simulink library "Surface_Profile_Axle2_zx_LR"  (R2025a)
settings: Solver=VariableStepAuto  StartTime=0.0  StopTime=10.0  RelTol=1e-3
Description:
  | Simscape Vehicle Templates Library
  | 
  | Copyright 2018-2025 The MathWorks, Inc.
settings Model: Creator=smiller  LastModifiedBy=smiller
settings ModelReferenceCC: EnableRefExpFcnMdlSchedulingChecks=on
settings RTWCC: GPUComputeCapability=3.5

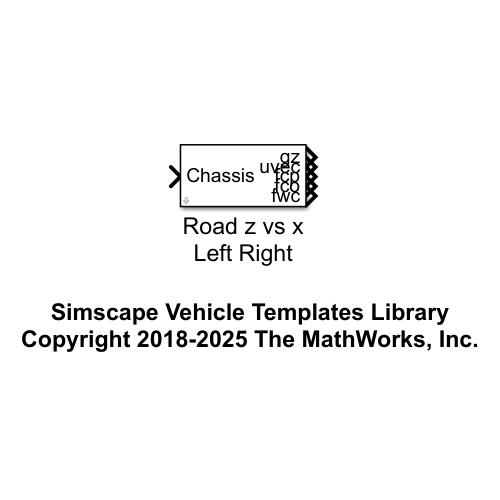
[thumbnail: Simulink's stored preview of the top-level diagram]
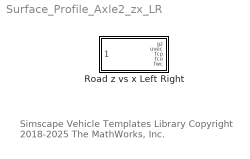
== system Surface_Profile_Axle2_zx_LR ==
  note: Simscape Vehicle Templates Library
      | Copyright 2018-2025 The MathWorks, Inc.
  Road z vs x Left Right : Subsystem  VariantControl=Rough_Road  mask{dist_x_l=flipud(Scene.RDF_Rough_Road.Road.extr_data_L(1330:end,1)), height_z_l=flipud(Scene.RDF_Rough_Road.Road.extr_data_L(1330:end,2)), dist_x_r=flipud(Scene.RDF_Rough_Road.Road.extr_data_R(1330:end,1)), height_z_r=flipud(Scene.RDF_Rough_Road.Road.extr_data_R(1330:end,2))}
      mask prompts: dist_x_l "Distance Vector Left [x] (m)"; height_z_l "Height Vector Left [z] (m)"; dist_x_r "Distance Vector Right [x] (m)"; height_z_r "Height Vector Right [z] (m)"
      mask init:
      | pitch_l = atan2(circshift(height_z_l,-2)-circshift(height_z_l,2),circshift(dist_x_l,-2)-circshift(dist_x_l,2));
      | pitch_l(1:2) = pitch_l(3);
      | pitch_l(end-1:end) = pitch_l(end-2);
      | 
      | pitch_r = atan2(circshift(height_z_r,-2)-circshift(height_z_r,2),circshift(dist_x_r,-2)-circshift(dist_x_r,2));
      | pitch_r(1:2) = pitch_r(3);
      | pitch_r(end-1:end) = pitch_r(end-2);

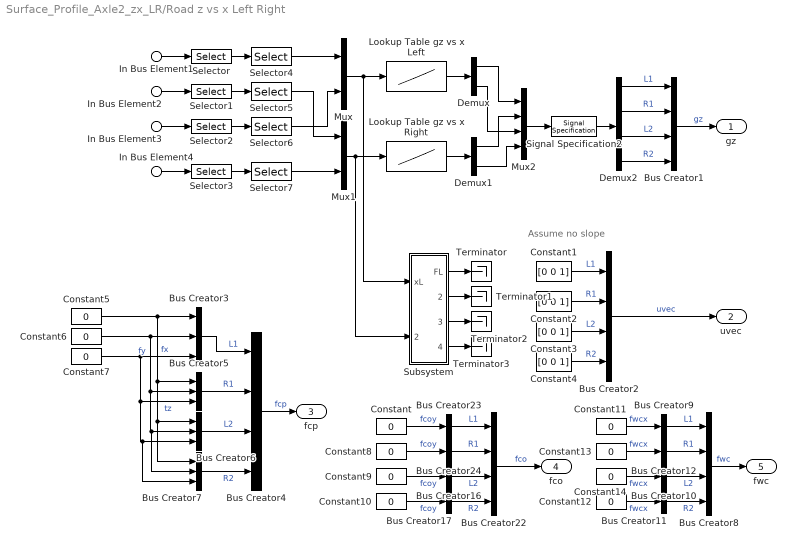
== system Surface_Profile_Axle2_zx_LR/Road z vs x Left Right ==
  note: Assume no slope
  In Bus Element1 : Inport  PortName=Chassis  Element=WhlL1.xyz
  In Bus Element2 : Inport  PortName=Chassis  Element=WhlR1.xyz
  In Bus Element3 : Inport  PortName=Chassis  Element=WhlL2.xyz
  In Bus Element4 : Inport  PortName=Chassis  Element=WhlR2.xyz
  Bus Creator{1..2,4,8,22} (5 alike) : BusCreator  Inputs=4
  Bus Creator{9..12,16..17,23..24} (8 alike) : BusCreator  Inputs=1
  Bus Creator{3,5..7} (4 alike) : BusCreator  Inputs=3
  Constant{,5..14} (11 alike) : Constant  Value=0
  Constant{1..4} (4 alike) : Constant  Value=[0 0 1]
  Demux : Demux  Outputs=2
  Demux1 : Demux  Outputs=2
  Demux2 : Demux
  Lookup Table gz vs x Left : Lookup_n-D  NumberOfTableDimensions=1  BreakpointsForDimension1=dist_x_l  Table=height_z_l  InternalRulePriority=Speed  RndMeth=Simplest
  Lookup Table gz vs x Right : Lookup_n-D  NumberOfTableDimensions=1  BreakpointsForDimension1=dist_x_r  Table=height_z_r  InternalRulePriority=Speed  RndMeth=Simplest
  Mux : Mux  Inputs=2
  Mux1 : Mux  Inputs=2
  Mux2 : Mux
  Selector{,1..3} (4 alike) : Selector  InputPortWidth=3  IndexOptions=Index vector (dialog)  Indices=[1 2]  OutputSizes=1
  Selector{4..7} (4 alike) : Selector  InputPortWidth=2  IndexOptions=Index vector (dialog)  Indices=1  OutputSizes=1
  Signal Specification2 : SignalSpecification  Unit=m
  Subsystem : Subsystem
  Terminator{,1..3} (4 alike) : Terminator
  gz : Outport  VectorParamsAs1DForOutWhenUnconnected=off
  uvec : Outport  Port=2  VectorParamsAs1DForOutWhenUnconnected=off
  fcp : Outport  Port=3  VectorParamsAs1DForOutWhenUnconnected=off
  fco : Outport  Port=4  VectorParamsAs1DForOutWhenUnconnected=off
  fwc : Outport  Port=5  VectorParamsAs1DForOutWhenUnconnected=off
  wires:
  Constant7/1 -> Bus Creator3/3, Bus Creator5/3, Bus Creator6/3, Bus Creator7/3  "tz"
  Constant6/1 -> Bus Creator3/2, Bus Creator5/2, Bus Creator6/2, Bus Creator7/2  "fy"
  Constant5/1 -> Bus Creator3/1, Bus Creator5/1, Bus Creator6/1, Bus Creator7/1  "fx"
  Bus Creator7/1 -> Bus Creator4/4  "R2"
  Bus Creator6/1 -> Bus Creator4/3  "L2"
  Bus Creator3/1 -> Bus Creator4/1  "L1"
  Bus Creator5/1 -> Bus Creator4/2  "R1"
  Bus Creator4/1 -> fcp/1  "fcp"
  Subsystem/3(RL) -> Terminator2/1
  Subsystem/2(FR) -> Terminator1/1
  Subsystem/4(RR) -> Terminator3/1
  Subsystem/1(FL) -> Terminator/1
  Constant4/1 -> Bus Creator2/4  "R2"
  Bus Creator2/1 -> uvec/1  "uvec"
  Constant2/1 -> Bus Creator2/2  "R1"
  Constant3/1 -> Bus Creator2/3  "L2"
  Constant1/1 -> Bus Creator2/1  "L1"
  Bus Creator1/1 -> gz/1  "gz"
  Demux2/4 -> Bus Creator1/4  "R2"
  Demux2/3 -> Bus Creator1/3  "L2"
  Demux2/2 -> Bus Creator1/2  "R1"
  Demux2/1 -> Bus Creator1/1  "L1"
  Mux/1 -> Lookup Table gz vs x Left/1, Subsystem/1(xL)
  Mux1/1 -> Lookup Table gz vs x Right/1, Subsystem/2(xR)
  Mux2/1 -> Signal Specification2/1
  Demux1/2 -> Mux2/4
  Demux/2 -> Mux2/3
  Demux1/1 -> Mux2/2
  Demux/1 -> Mux2/1
  Lookup Table gz vs x Left/1 -> Demux/1
  Lookup Table gz vs x Right/1 -> Demux1/1
  Selector4/1 -> Mux/1
  Selector5/1 -> Mux1/1
  Selector6/1 -> Mux/2
  Selector7/1 -> Mux1/2
  Selector3/1 -> Selector7/1
  Selector2/1 -> Selector6/1
  Selector1/1 -> Selector5/1
  Selector/1 -> Selector4/1
  In Bus Element4/1 -> Selector3/1
  In Bus Element2/1 -> Selector1/1
  In Bus Element1/1 -> Selector/1
  In Bus Element3/1 -> Selector2/1
  Signal Specification2/1 -> Demux2/1
  Bus Creator22/1 -> fco/1  "fco"
  Bus Creator23/1 -> Bus Creator22/1  "L1"
  Bus Creator17/1 -> Bus Creator22/4  "R2"
  Constant14/1 -> Bus Creator10/1  "fwcx"
  Constant13/1 -> Bus Creator12/1  "fwcx"
  Bus Creator8/1 -> fwc/1  "fwc"
  Constant10/1 -> Bus Creator17/1  "fcoy"
  Bus Creator11/1 -> Bus Creator8/4  "R2"
  Bus Creator9/1 -> Bus Creator8/1  "L1"
  Bus Creator16/1 -> Bus Creator22/3  "L2"
  Bus Creator10/1 -> Bus Creator8/3  "L2"
  Constant/1 -> Bus Creator23/1  "fcoy"
  Bus Creator24/1 -> Bus Creator22/2  "R1"
  Bus Creator12/1 -> Bus Creator8/2  "R1"
  Constant11/1 -> Bus Creator9/1  "fwcx"
  Constant9/1 -> Bus Creator16/1  "fcoy"
  Constant12/1 -> Bus Creator11/1  "fwcx"
  Constant8/1 -> Bus Creator24/1  "fcoy"

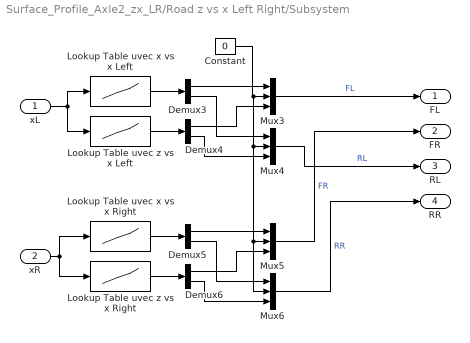
== system Surface_Profile_Axle2_zx_LR/Road z vs x Left Right/Subsystem ==
  xL : Inport
  xR : Inport  Port=2
  Constant : Constant  Value=0
  Demux{3..6} (4 alike) : Demux  Outputs=2
  Lookup Table uvec x vs x Left : Lookup_n-D  NumberOfTableDimensions=1  BreakpointsForDimension1=dist_x_l  Table=sin(pitch_l)  InternalRulePriority=Speed  RndMeth=Simplest
  Lookup Table uvec x vs x Right : Lookup_n-D  NumberOfTableDimensions=1  BreakpointsForDimension1=dist_x_r  Table=sin(pitch_r)  InternalRulePriority=Speed  RndMeth=Simplest
  Lookup Table uvec z vs x Left : Lookup_n-D  NumberOfTableDimensions=1  BreakpointsForDimension1=dist_x_l  Table=cos(pitch_l)  InternalRulePriority=Speed  RndMeth=Simplest
  Lookup Table uvec z vs x Right : Lookup_n-D  NumberOfTableDimensions=1  BreakpointsForDimension1=dist_x_r  Table=cos(pitch_r)  InternalRulePriority=Speed  RndMeth=Simplest
  Mux{3..6} (4 alike) : Mux  Inputs=3
  FL : Outport  VectorParamsAs1DForOutWhenUnconnected=off
  FR : Outport  Port=2  VectorParamsAs1DForOutWhenUnconnected=off
  RL : Outport  Port=3  VectorParamsAs1DForOutWhenUnconnected=off
  RR : Outport  Port=4  VectorParamsAs1DForOutWhenUnconnected=off
  wires:
  Mux4/1 -> RL/1  "RL"
  Lookup Table uvec x vs x Right/1 -> Demux5/1
  Demux5/1 -> Mux5/1
  Demux6/1 -> Mux5/3
  Demux5/2 -> Mux6/1
  Mux5/1 -> FR/1  "FR"
  Constant/1 -> Mux3/2, Mux4/2, Mux6/2, Mux5/2
  Demux4/2 -> Mux4/3
  Lookup Table uvec z vs x Right/1 -> Demux6/1
  Demux3/1 -> Mux3/1
  Demux3/2 -> Mux4/1
  Lookup Table uvec z vs x Left/1 -> Demux4/1
  xR/1 -> Lookup Table uvec z vs x Right/1, Lookup Table uvec x vs x Right/1
  Demux6/2 -> Mux6/3
  Mux3/1 -> FL/1  "FL"
  Demux4/1 -> Mux3/3
  Mux6/1 -> RR/1  "RR"
  xL/1 -> Lookup Table uvec z vs x Left/1, Lookup Table uvec x vs x Left/1
  Lookup Table uvec x vs x Left/1 -> Demux3/1
